simulink model "Plant"  (R2019b)
settings: Solver=VariableStepAuto  StartTime=0.0  StopTime=10.0  RelTol=1e-3
settings Model: Creator=Lightning  LastModifiedBy=Lightning

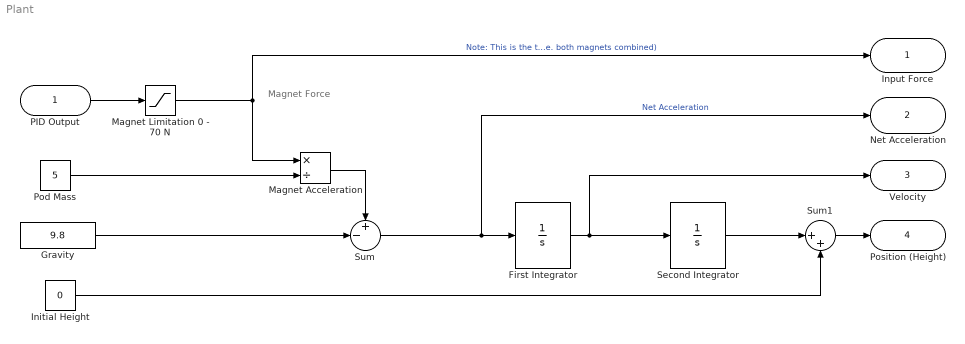
== system Plant ==
  note: Magnet
      |  Force
  PID Output : Inport
  First Integrator : Integrator
  Gravity : Constant  Value=9.8
  Initial Height : Constant  Value=0
  Magnet Acceleration : Product  Inputs=*/
  Magnet Limitation 0 - 70 N : Saturate  UpperLimit=70  LowerLimit=0
  Pod Mass : Constant  Value=5
  Second Integrator : Integrator
  Sum : Sum  Inputs=+-|
  Sum1 : Sum  Inputs=|++
  Input Force : Outport
  Net Acceleration : Outport  Port=2
  "Velocity " : Outport  Port=3
  Position (Height) : Outport  Port=4
  wires:
  First Integrator/1 -> Second Integrator/1, "Velocity "/1
  Second Integrator/1 -> Sum1/1
  Magnet Limitation 0 - 70 N/1 -> Input Force/1, Magnet Acceleration/1  "Note: This is the total force on the pod from the magnets (i.e. both magnets combined)"
  Pod Mass/1 -> Magnet Acceleration/2
  Gravity/1 -> Sum/2
  Magnet Acceleration/1 -> Sum/1
  Sum/1 -> Net Acceleration/1, First Integrator/1  "Net Acceleration"
  Sum1/1 -> Position (Height)/1
  Initial Height/1 -> Sum1/2
  PID Output/1 -> Magnet Limitation 0 - 70 N/1
